simulink library "AC"  (R2020b)
settings: Solver=VariableStepAuto  StartTime=0.0  StopTime=10.0  RelTol=1e-3
undefined symbols (not defined in the file or in its folder): entity, initX, instancedAC, m, n, WP, WPabort, WPspeed
libraries: aerolibactuator x6, $bdroot x1
settings Model: Creator=Rafael.Casado  LastModifiedBy=usuario
settings DataIOCC: ReturnWorkspaceOutputs=off
settings DebuggingCC: ArithmeticOperatorsInVariantConditions=warning
settings SFSimCC: SimUseLocalCustomCode=off  CustomCodeUndefinedFunction=UseInterfaceOnly
settings RTWCC: RTWUseLocalCustomCode=off
settings CodeAppCC: StateflowObjectComments=on

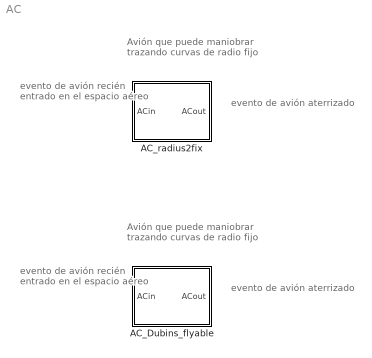
== system AC ==
  note: Avión que puede maniobrar trazando curvas de radio fijo
  note: evento de avión aterrizado
  note: evento de avión recién entrado en el espacio aéreo
  note: Avión que puede maniobrar trazando curvas de radio fijo
  note: evento de avión aterrizado
  note: evento de avión recién entrado en el espacio aéreo
  AC_Dubins_flyable : Subsystem
  AC_radius2fix : Subsystem

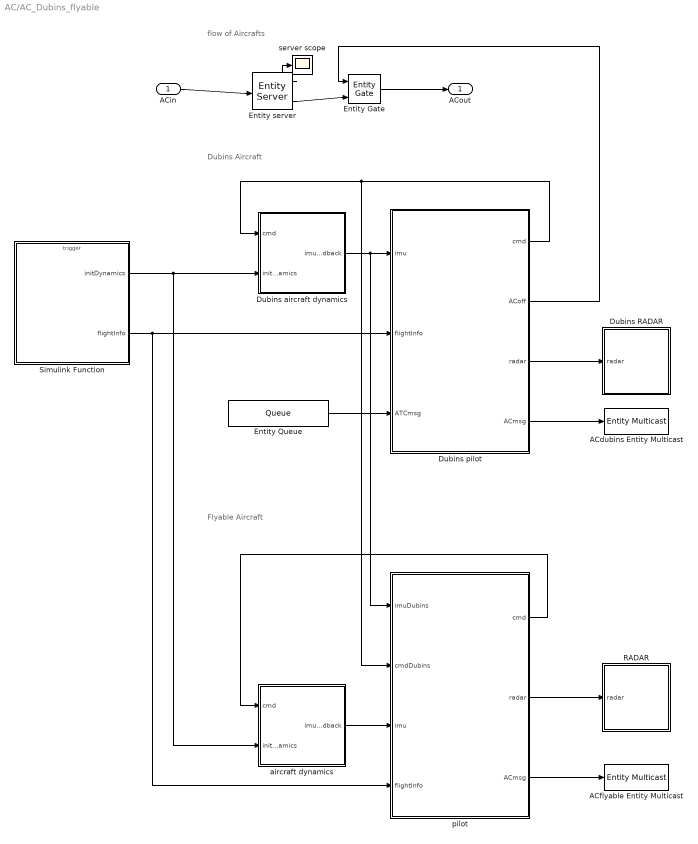
== system AC/AC_Dubins_flyable ==
  note: Dubins Aircraft
  note: flow of Aircrafts
  note: Flyable Aircraft
  ACin : Inport
  ACdubins Entity Multicast : EntityMulticast  InputPortMessageModes=m  MulticastTag=ACcomm
  ACflyable Entity Multicast : EntityMulticast  InputPortMessageModes=m  MulticastTag=ACcomm
  Dubins RADAR : Subsystem
      mask Display:
      | plot([00 10], [05 05])
      | plot([05 05], [00 10])
      | 
      | plot([01 09 09 01 01], [01 01 09 09 01])
      | plot([03 07 07 03 03], [03 03 07 07 03])
  Dubins aircraft dynamics : Subsystem
      mask Display:
      | patch([50 -50 -50 50], [40 40 -60 -60], [1 1 1])
      | 
      | patch([8 -8 -8 8], [6 6 -6 -6], [0.7 0.7 0.7])
      | 
      | patch([ 8  8  28  28], [0 -2 2 4], [0.5 0.5 0.5])
      | patch([-8 -8 -28 -28], [0 -2 2 4], [0.5 0.5 0.5])
      | 
      | patch([1 0 -1], [6 18 6], [0.5 0.5 0.5])
  Dubins pilot : Stateflow chart  TreatAsAtomicUnit=on
  Entity Gate : EntityGate  InputPortMessageModes=m,m  OutputPortMessageModes=m  OperatingMode=Release gate
  Entity Queue : Queue  OutputPortMessageModes=m  Capacity=100  EntityArrivalSource=Multicast  MulticastTag=ATCcomm
  Entity server : EntityServer  InputPortMessageModes=m  OutputPortMessageModes=n,m  Capacity=1  ServiceTimeValue=10  EntryAction=instancedAC(entity.flightId,true);  ServiceCompleteAction=instancedAC(entity.flightId,false);  NumberEntitiesInBlock=on
      settings: OutputPortMap=o1,o9
  RADAR : Subsystem
      mask Display:
      | plot([00 10], [05 05])
      | plot([05 05], [00 10])
      | 
      | plot([01 09 09 01 01], [01 01 09 09 01])
      | plot([03 07 07 03 03], [03 03 07 07 03])
  Simulink Function : Subsystem  TreatAsAtomicUnit=on
  aircraft dynamics : Subsystem
      mask Display:
      | patch([50 -50 -50 50], [40 40 -60 -60], [1 1 1])
      | 
      | patch([8 -8 -8 8], [6 6 -6 -6], [0.7 0.7 0.7])
      | 
      | patch([ 8  8  28  28], [0 -2 2 4], [0.5 0.5 0.5])
      | patch([-8 -8 -28 -28], [0 -2 2 4], [0.5 0.5 0.5])
      | 
      | patch([1 0 -1], [6 18 6], [0.5 0.5 0.5])
  pilot : Stateflow chart  TreatAsAtomicUnit=on
  server scope : Scope
  ACout : Outport  VectorParamsAs1DForOutWhenUnconnected=off
  wires:
  Simulink Function/2(flightInfo) -> pilot/4(flightInfo), Dubins pilot/2(flightInfo)
  ACin/1 -> Entity server/1
  Dubins aircraft dynamics/1(imu_feedback) -> Dubins pilot/1(imu), pilot/1(imuDubins)
  pilot/1(cmd) -> aircraft dynamics/1(cmd)
  Dubins pilot/2(ACoff) -> Entity Gate/1
  pilot/2(radar) -> RADAR/1(radar)
  Simulink Function/1(initDynamics) -> aircraft dynamics/2(initDynamics), Dubins aircraft dynamics/2(initDynamics)
  Dubins pilot/1(cmd) -> pilot/2(cmdDubins), Dubins aircraft dynamics/1(cmd)
  Entity server/1 -> server scope/1
  Dubins pilot/3(radar) -> Dubins RADAR/1(radar)
  aircraft dynamics/1(imu_feedback) -> pilot/3(imu)
  Dubins pilot/4(ACmsg) -> ACdubins Entity Multicast/1
  Entity Gate/1 -> ACout/1
  Entity server/2 -> Entity Gate/2
  Entity Queue/1 -> Dubins pilot/3(ATCmsg)
  pilot/3(ACmsg) -> ACflyable Entity Multicast/1

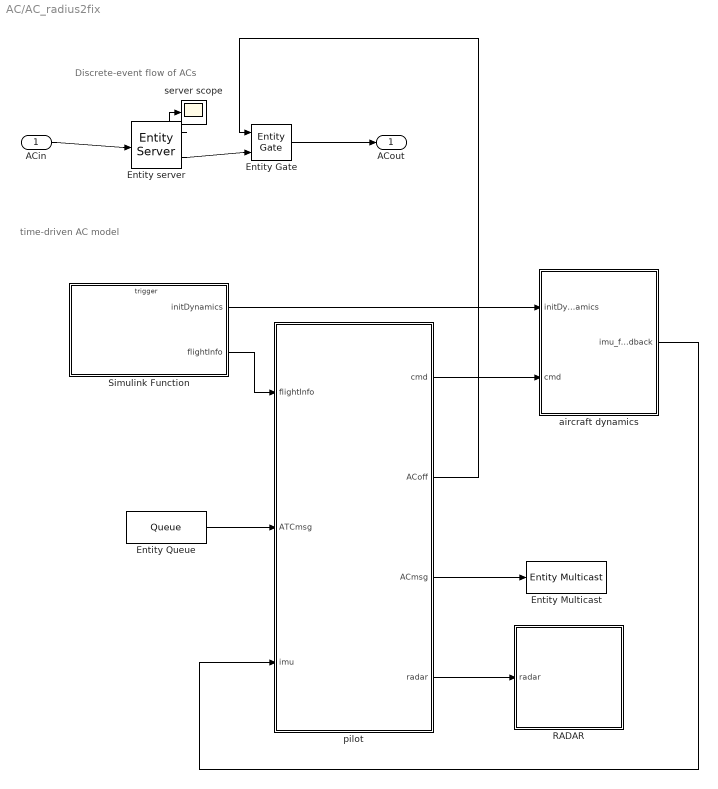
== system AC/AC_radius2fix ==
  note: Discrete-event flow of ACs
  note: time-driven AC model
  ACin : Inport
  Entity Gate : EntityGate  InputPortMessageModes=m,m  OutputPortMessageModes=m  OperatingMode=Release gate
  Entity Multicast : EntityMulticast  InputPortMessageModes=m  MulticastTag=ACcomm
  Entity Queue : Queue  OutputPortMessageModes=m  Capacity=100  EntityArrivalSource=Multicast  MulticastTag=ATCcomm
  Entity server : EntityServer  InputPortMessageModes=m  OutputPortMessageModes=n,m  Capacity=1  ServiceTimeValue=10  EntryAction=instancedAC(entity.flightId,true);  ServiceCompleteAction=instancedAC(entity.flightId,false);  NumberEntitiesInBlock=on
      settings: OutputPortMap=o1,o9
  RADAR : Subsystem
      mask Display:
      | plot([00 10], [05 05])
      | plot([05 05], [00 10])
      | 
      | plot([01 09 09 01 01], [01 01 09 09 01])
      | plot([03 07 07 03 03], [03 03 07 07 03])
  Simulink Function : Subsystem  TreatAsAtomicUnit=on
  aircraft dynamics : Subsystem
      mask Display:
      | patch([50 -50 -50 50], [40 40 -60 -60], [1 1 1])
      | 
      | patch([8 -8 -8 8], [6 6 -6 -6], [0.7 0.7 0.7])
      | 
      | patch([ 8  8  28  28], [0 -2 2 4], [0.5 0.5 0.5])
      | patch([-8 -8 -28 -28], [0 -2 2 4], [0.5 0.5 0.5])
      | 
      | patch([1 0 -1], [6 18 6], [0.5 0.5 0.5])
  pilot : Stateflow chart  TreatAsAtomicUnit=on
  server scope : Scope
  ACout : Outport  VectorParamsAs1DForOutWhenUnconnected=off
  wires:
  aircraft dynamics/1(imu_feedback) -> pilot/3(imu)
  Simulink Function/1(initDynamics) -> aircraft dynamics/1(initDynamics)
  ACin/1 -> Entity server/1
  Simulink Function/2(flightInfo) -> pilot/1(flightInfo)
  Entity Gate/1 -> ACout/1
  Entity server/2 -> Entity Gate/2
  pilot/2(ACoff) -> Entity Gate/1
  pilot/1(cmd) -> aircraft dynamics/2(cmd)
  Entity server/1 -> server scope/1
  pilot/4(radar) -> RADAR/1(radar)
  Entity Queue/1 -> pilot/2(ATCmsg)
  pilot/3(ACmsg) -> Entity Multicast/1

== system AC/AC_Dubins_flyable/Dubins RADAR ==
  radar : Inport
  RADAR figure : MATLABFcn  Commented=on  StartFcn=|  MATLABFcn=PBNsim_RADAR  OutputDimensions=0  Output1D=off
      | clear functions;
      | clc;
      mask Display: patch([50 -50 -50 50], [40 40 -60 -60], [1 1 1])
  virtual bus : Subsystem
  wires:
  radar/1 -> virtual bus/1(nvbus)
  virtual bus/1(vbus) -> RADAR figure/1

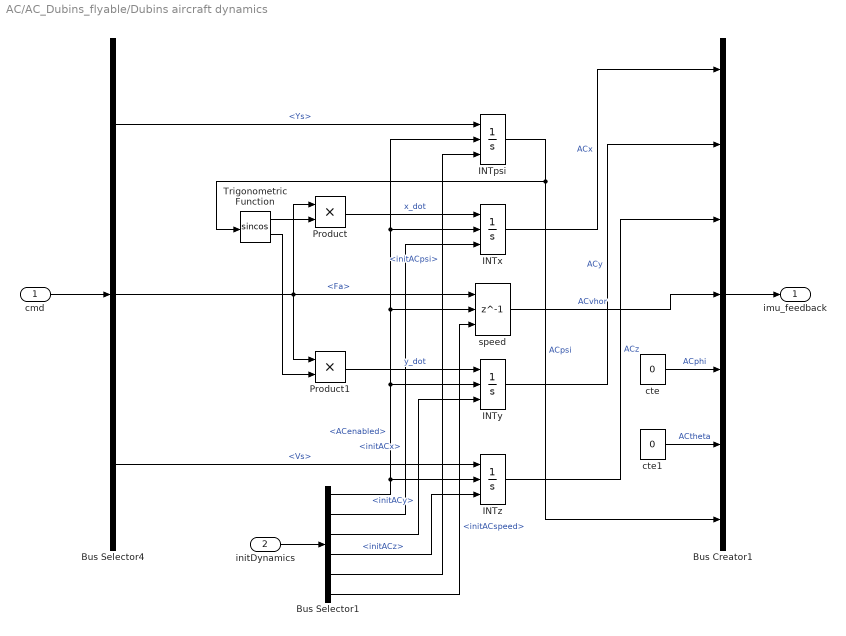
== system AC/AC_Dubins_flyable/Dubins aircraft dynamics ==
  cmd : Inport
  initDynamics : Inport  Port=2
  Bus Creator1 : BusCreator  Inputs=7  OutDataTypeStr=Bus: bus_IMU
      settings: InheritFromInputs=off
  Bus Selector1 : BusSelector  OutputSignals=ACenabled,initACx,initACy,initACz,initACpsi,initACspeed
  Bus Selector4 : BusSelector  OutputSignals=Ys,Fa,Vs
  INTpsi : Integrator  ExternalReset=rising  InitialConditionSource=external  InitialCondition=initX(3)
  INTx : Integrator  ExternalReset=rising  InitialConditionSource=external  InitialCondition=initX(3)
  INTy : Integrator  ExternalReset=rising  InitialConditionSource=external  InitialCondition=initX(3)
  INTz : Integrator  ExternalReset=rising  InitialConditionSource=external  InitialCondition=initX(3)
  Product : Product
  Product1 : Product
  Trigonometric Function : Trigonometry  Operator=sincos
  cte : Constant  Value=0
  cte1 : Constant  Value=0
  speed : Delay  DelayLength=1  InitialConditionSource=Input port  InitialCondition=convvel(240,'kts','m/s');  ExternalReset=Rising
      settings: InputPortMap=u0,r5,p4
  imu_feedback : Outport  SourceOfInitialOutputValue=Input signal  OutputWhenDisabled=reset  VectorParamsAs1DForOutWhenUnconnected=off
  wires:
  Bus Selector4/2 -> Product/1, speed/1, Product1/1  "<Fa>"
  Trigonometric Function/1 -> Product/2
  Product1/1 -> INTy/1  "y_dot"
  Product/1 -> INTx/1  "x_dot"
  Trigonometric Function/2 -> Product1/2
  Bus Selector4/3 -> INTz/1  "<Vs>"
  cmd/1 -> Bus Selector4/1
  Bus Selector4/1 -> INTpsi/1  "<Ys>"
  cte1/1 -> Bus Creator1/6  "ACtheta"
  INTz/1 -> Bus Creator1/3  "ACz"
  INTx/1 -> Bus Creator1/1  "ACx"
  cte/1 -> Bus Creator1/5  "ACphi"
  INTy/1 -> Bus Creator1/2  "ACy"
  Bus Creator1/1 -> imu_feedback/1
  initDynamics/1 -> Bus Selector1/1
  Bus Selector1/2 -> INTx/3  "<initACx>"
  Bus Selector1/3 -> INTy/3  "<initACy>"
  Bus Selector1/4 -> INTz/3  "<initACz>"
  Bus Selector1/5 -> INTpsi/3  "<initACpsi>"
  Bus Selector1/1 -> INTz/2, speed/2, INTpsi/2, INTx/2, INTy/2  "<ACenabled>"
  INTpsi/1 -> Bus Creator1/7, Trigonometric Function/1  "ACpsi"
  speed/1 -> Bus Creator1/4  "ACvhor"
  Bus Selector1/6 -> speed/3  "<initACspeed>"

== system AC/AC_Dubins_flyable/RADAR ==
  radar : Inport
  RADAR figure : MATLABFcn  StartFcn=|  MATLABFcn=PBNsim_RADAR  OutputDimensions=0  Output1D=off
      | clear functions;
      | clc;
      mask Display: patch([50 -50 -50 50], [40 40 -60 -60], [1 1 1])
  virtual bus : $bdroot/AC_Dubins_flyable/Dubins RADAR/virtual bus  SystemSampleTime=-1  VariantActivationTime=update diagram  Latency=0  AutoFrameSizeCalculation=off
  wires:
  radar/1 -> virtual bus/1
  virtual bus/1 -> RADAR figure/1

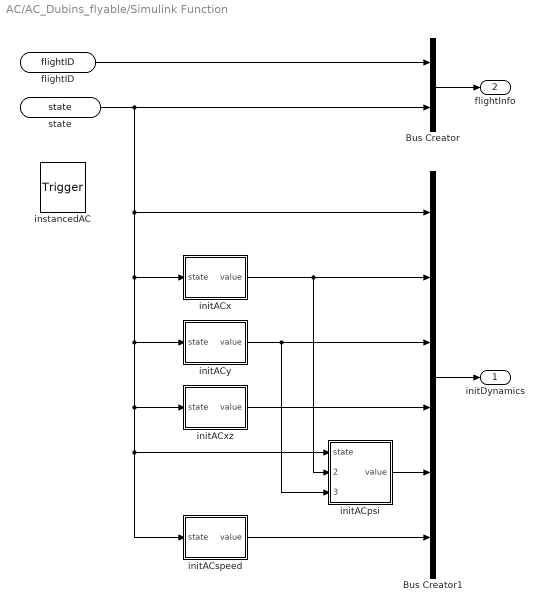
== system AC/AC_Dubins_flyable/Simulink Function ==
  instancedAC : TriggerPort  TriggerType=function-call  IsSimulinkFunction=on  FunctionName=instancedAC  FunctionVisibility=scoped  VariantControl=Variant
  Bus Creator : BusCreator  Inputs=2  OutDataTypeStr=Bus: bus_ADSB
      settings: InheritFromInputs=off
  Bus Creator1 : BusCreator  Inputs=6  OutDataTypeStr=Bus: bus_initDynamics
      settings: InheritFromInputs=off
  initACpsi : Subsystem
  initACspeed : Subsystem
  initACx : Subsystem
  initACxz : Subsystem
  initACy : Subsystem
  flightID : ArgIn  ArgumentName=flightID
  state : ArgIn  Port=2  OutDataTypeStr=boolean  ArgumentName=state
  initDynamics : Outport  VectorParamsAs1DForOutWhenUnconnected=off
  flightInfo : Outport  Port=2  VectorParamsAs1DForOutWhenUnconnected=off
  wires:
  state/1 -> initACy/1(state), initACxz/1(state), initACpsi/1(state), initACspeed/1(state), initACx/1(state), Bus Creator1/1, Bus Creator/2
  Bus Creator/1 -> flightInfo/1
  flightID/1 -> Bus Creator/1
  Bus Creator1/1 -> initDynamics/1
  initACx/1(value) -> initACpsi/2(initACx), Bus Creator1/2
  initACy/1(value) -> initACpsi/3(initACy), Bus Creator1/3
  initACxz/1(value) -> Bus Creator1/4
  initACpsi/1(value) -> Bus Creator1/5
  initACspeed/1(value) -> Bus Creator1/6

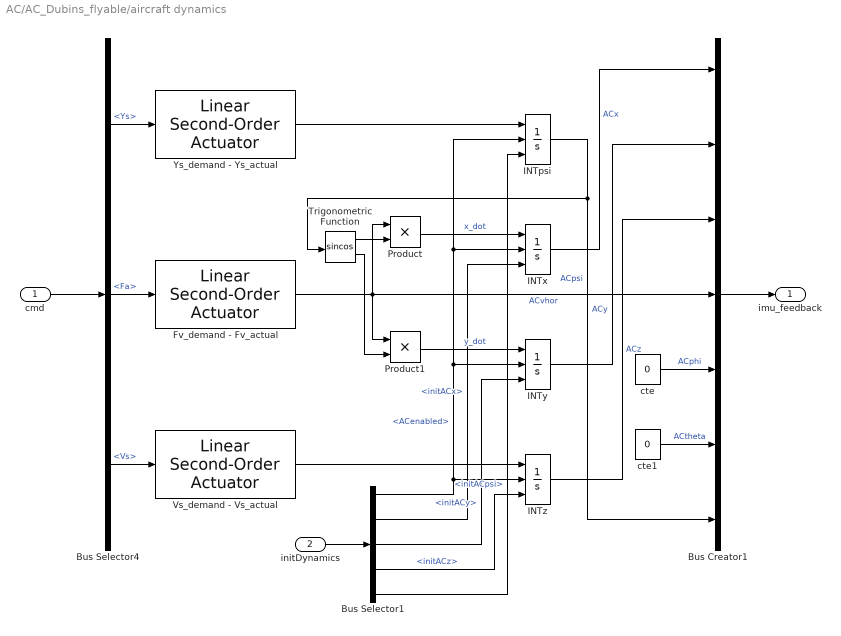
== system AC/AC_Dubins_flyable/aircraft dynamics ==
  cmd : Inport
  initDynamics : Inport  Port=2
  Bus Creator1 : BusCreator  Inputs=7  OutDataTypeStr=Bus: bus_IMU
      settings: InheritFromInputs=off
  Bus Selector1 : BusSelector  OutputSignals=ACenabled,initACx,initACy,initACz,initACpsi
  Bus Selector4 : BusSelector  OutputSignals=Ys,Fa,Vs
  Fv_demand - Fv_actual : aerolibactuator/Linear Second-Order Actuator  wn_fin=0.6  z_fin=1  fin_act_0=convvel(240,'kts','m/s');  fin_act_vel=0
      settings: SourceProductBaseCode=AE
  INTpsi : Integrator  ExternalReset=rising  InitialConditionSource=external  InitialCondition=initX(3)
  INTx : Integrator  ExternalReset=rising  InitialConditionSource=external  InitialCondition=initX(3)
  INTy : Integrator  ExternalReset=rising  InitialConditionSource=external  InitialCondition=initX(3)
  INTz : Integrator  ExternalReset=rising  InitialConditionSource=external  InitialCondition=initX(3)
  Product : Product
  Product1 : Product
  Trigonometric Function : Trigonometry  Operator=sincos
  Vs_demand - Vs_actual : aerolibactuator/Linear Second-Order Actuator  wn_fin=0.6  z_fin=1  fin_act_0=0  fin_act_vel=0
      settings: SourceProductBaseCode=AE
  Ys_demand - Ys_actual : aerolibactuator/Linear Second-Order Actuator  wn_fin=0.8  z_fin=1  fin_act_0=0  fin_act_vel=0
      settings: SourceProductBaseCode=AE
  cte : Constant  Value=0
  cte1 : Constant  Value=0
  imu_feedback : Outport  SourceOfInitialOutputValue=Input signal  OutputWhenDisabled=reset  VectorParamsAs1DForOutWhenUnconnected=off
  wires:
  Bus Selector4/2 -> Fv_demand - Fv_actual/1  "<Fa>"
  Fv_demand - Fv_actual/1 -> Product/1, Product1/1, Bus Creator1/4  "ACvhor"
  Trigonometric Function/1 -> Product/2
  Product1/1 -> INTy/1  "y_dot"
  Product/1 -> INTx/1  "x_dot"
  Trigonometric Function/2 -> Product1/2
  Bus Selector4/3 -> Vs_demand - Vs_actual/1  "<Vs>"
  cmd/1 -> Bus Selector4/1
  Bus Selector4/1 -> Ys_demand - Ys_actual/1  "<Ys>"
  cte1/1 -> Bus Creator1/6  "ACtheta"
  INTz/1 -> Bus Creator1/3  "ACz"
  INTx/1 -> Bus Creator1/1  "ACx"
  cte/1 -> Bus Creator1/5  "ACphi"
  INTy/1 -> Bus Creator1/2  "ACy"
  Bus Creator1/1 -> imu_feedback/1
  initDynamics/1 -> Bus Selector1/1
  Bus Selector1/2 -> INTx/3  "<initACx>"
  Bus Selector1/3 -> INTy/3  "<initACy>"
  Bus Selector1/4 -> INTz/3  "<initACz>"
  Bus Selector1/5 -> INTpsi/3  "<initACpsi>"
  Bus Selector1/1 -> INTz/2, INTpsi/2, INTx/2, INTy/2  "<ACenabled>"
  INTpsi/1 -> Trigonometric Function/1, Bus Creator1/7  "ACpsi"
  Vs_demand - Vs_actual/1 -> INTz/1
  Ys_demand - Ys_actual/1 -> INTpsi/1

== system AC/AC_radius2fix/RADAR ==
  radar : Inport
  RADAR figure : MATLABFcn  StartFcn=|  MATLABFcn=PBNsim_RADAR  OutputDimensions=0  Output1D=off
      | clear functions;
      | clc;
      mask Display: patch([50 -50 -50 50], [40 40 -60 -60], [1 1 1])
  virtual bus : Subsystem
  wires:
  radar/1 -> virtual bus/1(nvbus)
  virtual bus/1(vbus) -> RADAR figure/1

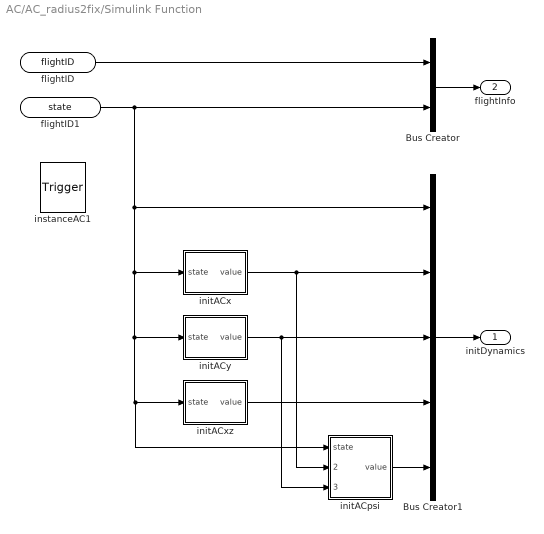
== system AC/AC_radius2fix/Simulink Function ==
  instanceAC1 : TriggerPort  TriggerType=function-call  IsSimulinkFunction=on  FunctionName=instancedAC  FunctionVisibility=scoped  VariantControl=Variant
  Bus Creator : BusCreator  Inputs=2  OutDataTypeStr=Bus: bus_ADSB
      settings: InheritFromInputs=off
  Bus Creator1 : BusCreator  Inputs=5  OutDataTypeStr=Bus: bus_initDynamics
      settings: InheritFromInputs=off
  initACpsi : Subsystem
  initACx : Subsystem
  initACxz : Subsystem
  initACy : Subsystem
  flightID : ArgIn  ArgumentName=flightID
  flightID1 : ArgIn  Port=2  OutDataTypeStr=boolean  ArgumentName=state
  initDynamics : Outport  VectorParamsAs1DForOutWhenUnconnected=off
  flightInfo : Outport  Port=2  VectorParamsAs1DForOutWhenUnconnected=off
  wires:
  initACpsi/1(value) -> Bus Creator1/5
  initACxz/1(value) -> Bus Creator1/4
  initACy/1(value) -> initACpsi/3(initACy), Bus Creator1/3
  initACx/1(value) -> Bus Creator1/2, initACpsi/2(initACx)
  Bus Creator1/1 -> initDynamics/1
  flightID/1 -> Bus Creator/1
  Bus Creator/1 -> flightInfo/1
  flightID1/1 -> Bus Creator/2, initACx/1(state), initACxz/1(state), initACpsi/1(state), initACy/1(state), Bus Creator1/1

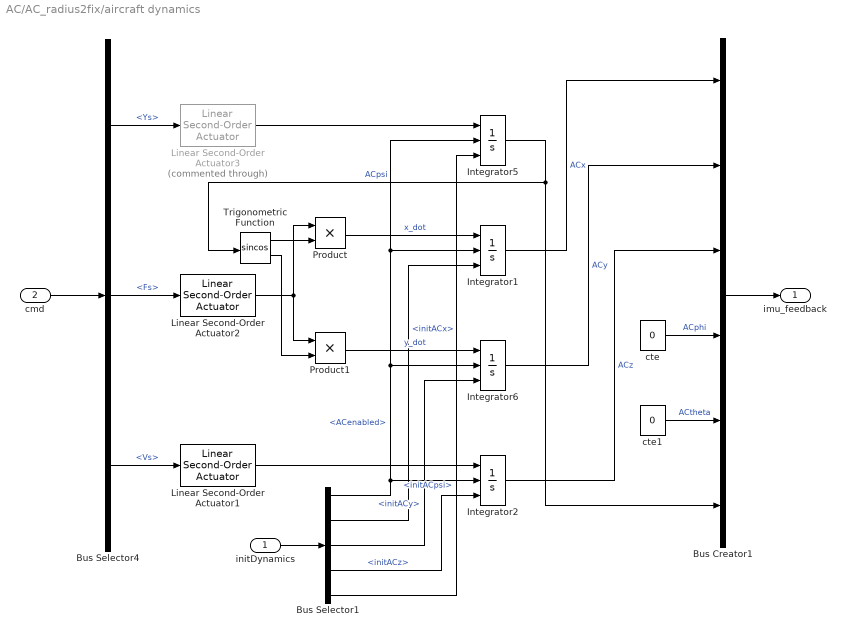
== system AC/AC_radius2fix/aircraft dynamics ==
  initDynamics : Inport
  cmd : Inport  Port=2
  Bus Creator1 : BusCreator  Inputs=6  OutDataTypeStr=Bus: bus_IMU
      settings: InheritFromInputs=off
  Bus Selector1 : BusSelector  OutputSignals=ACenabled,initACx,initACy,initACz,initACpsi
  Bus Selector4 : BusSelector  OutputSignals=Ys,Fs,Vs
  Integrator{1..2,5..6} (4 alike) : Integrator  ExternalReset=rising  InitialConditionSource=external  InitialCondition=initX(3)
  Linear Second-Order Actuator1 : aerolibactuator/Linear Second-Order Actuator  wn_fin=1  z_fin=1  fin_act_0=0  fin_act_vel=0
      settings: SourceProductBaseCode=AE
  Linear Second-Order Actuator2 : aerolibactuator/Linear Second-Order Actuator  wn_fin=1  z_fin=1  fin_act_0=convvel(240,'kts','m/s');  fin_act_vel=0
      settings: SourceProductBaseCode=AE
  Linear Second-Order Actuator3 : aerolibactuator/Linear Second-Order Actuator  Commented=through  wn_fin=1  z_fin=1  fin_act_0=0  fin_act_vel=0
      settings: SourceProductBaseCode=AE
  Product : Product
  Product1 : Product
  Trigonometric Function : Trigonometry  Operator=sincos
  cte : Constant  Value=0
  cte1 : Constant  Value=0
  imu_feedback : Outport  SourceOfInitialOutputValue=Input signal  OutputWhenDisabled=reset  VectorParamsAs1DForOutWhenUnconnected=off
  wires:
  Integrator5/1 -> Bus Creator1/6, Trigonometric Function/1  "ACpsi"
  Bus Selector1/1 -> Integrator2/2, Integrator6/2, Integrator1/2, Integrator5/2  "<ACenabled>"
  Bus Selector1/5 -> Integrator5/3  "<initACpsi>"
  Bus Selector1/4 -> Integrator2/3  "<initACz>"
  Bus Selector1/3 -> Integrator6/3  "<initACy>"
  Bus Selector1/2 -> Integrator1/3  "<initACx>"
  initDynamics/1 -> Bus Selector1/1
  Bus Creator1/1 -> imu_feedback/1
  Integrator6/1 -> Bus Creator1/2  "ACy"
  cte/1 -> Bus Creator1/4  "ACphi"
  Integrator1/1 -> Bus Creator1/1  "ACx"
  Integrator2/1 -> Bus Creator1/3  "ACz"
  cte1/1 -> Bus Creator1/5  "ACtheta"
  Bus Selector4/1 -> Linear Second-Order Actuator3/1  "<Ys>"
  cmd/1 -> Bus Selector4/1
  Bus Selector4/3 -> Linear Second-Order Actuator1/1  "<Vs>"
  Trigonometric Function/2 -> Product1/2
  Product/1 -> Integrator1/1  "x_dot"
  Bus Selector4/2 -> Linear Second-Order Actuator2/1  "<Fs>"
  Product1/1 -> Integrator6/1  "y_dot"
  Trigonometric Function/1 -> Product/2
  Linear Second-Order Actuator2/1 -> Product/1, Product1/1
  Linear Second-Order Actuator1/1 -> Integrator2/1
  Linear Second-Order Actuator3/1 -> Integrator5/1

== system AC/AC_Dubins_flyable/Dubins RADAR/virtual bus ==
  nvbus : Inport
  Bus Creator : BusCreator  Inputs=7  OutDataTypeStr=Bus: bus_radar
      settings: InheritFromInputs=off
  Bus Selector4 : BusSelector  OutputSignals=ACid,ACenabled,ACdubins,ACx,ACy,ACz,ACpsi
  vbus : Outport  VectorParamsAs1DForOutWhenUnconnected=off
  wires:
  Bus Selector4/1 -> Bus Creator/1  "<ACid>"
  Bus Selector4/4 -> Bus Creator/4  "<ACx>"
  Bus Selector4/6 -> Bus Creator/6  "<ACz>"
  Bus Selector4/5 -> Bus Creator/5  "<ACy>"
  Bus Selector4/2 -> Bus Creator/2  "<ACenabled>"
  nvbus/1 -> Bus Selector4/1
  Bus Creator/1 -> vbus/1
  Bus Selector4/3 -> Bus Creator/3  "<ACdubins>"
  Bus Selector4/7 -> Bus Creator/7  "<ACpsi>"

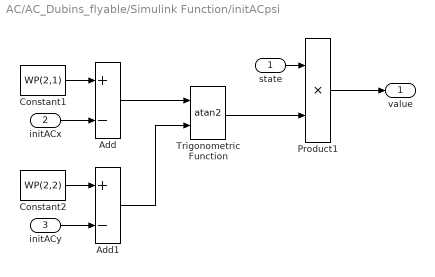
== system AC/AC_Dubins_flyable/Simulink Function/initACpsi ==
  state : Inport
  initACx : Inport  Port=2
  initACy : Inport  Port=3
  Add : Sum  Inputs=+-
  Add1 : Sum  Inputs=+-
  Constant1 : Constant  Value=WP(2,1)
  Constant2 : Constant  Value=WP(2,2)
  Product1 : Product
  Trigonometric Function : Trigonometry  Operator=atan2
  value : Outport  VectorParamsAs1DForOutWhenUnconnected=off
  wires:
  Add1/1 -> Trigonometric Function/2
  Add/1 -> Trigonometric Function/1
  Constant2/1 -> Add1/1
  initACy/1 -> Add1/2
  initACx/1 -> Add/2
  Constant1/1 -> Add/1
  state/1 -> Product1/1
  Trigonometric Function/1 -> Product1/2
  Product1/1 -> value/1

== system AC/AC_Dubins_flyable/Simulink Function/initACspeed ==
  state : Inport
  Add : Sum
  Constant1 : Constant  Value=convvel(WPspeed(2),'kts','m/s');
  Product1 : Product
  Uniform Random Number : UniformRandomNumber  Commented=on  Minimum=0  Maximum=100  Seed=randi(10000)
  value : Outport  VectorParamsAs1DForOutWhenUnconnected=off
  wires:
  Add/1 -> Product1/2
  Constant1/1 -> Add/1
  state/1 -> Product1/1
  Product1/1 -> value/1
  Uniform Random Number/1 -> Add/2

== system AC/AC_Dubins_flyable/Simulink Function/initACx ==
  state : Inport
  Add : Sum
  Constant1 : Constant  Value=WP(1,1)
  Product1 : Product
  Uniform Random Number : UniformRandomNumber  Commented=on  Minimum=0  Maximum=100  Seed=randi(10000)
  value : Outport  VectorParamsAs1DForOutWhenUnconnected=off
  wires:
  Add/1 -> Product1/2
  Constant1/1 -> Add/1
  state/1 -> Product1/1
  Product1/1 -> value/1
  Uniform Random Number/1 -> Add/2

== system AC/AC_Dubins_flyable/Simulink Function/initACxz ==
  state : Inport
  Add1 : Sum
  Constant2 : Constant  Value=WP(1,3)
  Product1 : Product
  Uniform Random Number1 : UniformRandomNumber  Commented=on  Minimum=0  Maximum=20  Seed=randi(10000)
  value : Outport  VectorParamsAs1DForOutWhenUnconnected=off
  wires:
  Uniform Random Number1/1 -> Add1/2
  Add1/1 -> Product1/2
  Constant2/1 -> Add1/1
  state/1 -> Product1/1
  Product1/1 -> value/1

== system AC/AC_Dubins_flyable/Simulink Function/initACy ==
  state : Inport
  Add2 : Sum
  Constant1 : Constant  Value=WP(1,2)
  Product1 : Product
  Uniform Random Number2 : UniformRandomNumber  Commented=on  Minimum=0  Maximum=100  Seed=randi(10000)
  value : Outport  VectorParamsAs1DForOutWhenUnconnected=off
  wires:
  Constant1/1 -> Add2/1
  Add2/1 -> Product1/2
  Uniform Random Number2/1 -> Add2/2
  state/1 -> Product1/1
  Product1/1 -> value/1

== system AC/AC_radius2fix/RADAR/virtual bus ==
  nvbus : Inport
  Bus Creator : BusCreator  Inputs=6  OutDataTypeStr=Bus: bus_radar
      settings: InheritFromInputs=off
  Bus Selector4 : BusSelector  OutputSignals=ACid,ACenabled,ACx,ACy,ACz,ACpsi
  vbus : Outport  VectorParamsAs1DForOutWhenUnconnected=off
  wires:
  Bus Creator/1 -> vbus/1
  nvbus/1 -> Bus Selector4/1
  Bus Selector4/2 -> Bus Creator/2  "<ACenabled>"
  Bus Selector4/4 -> Bus Creator/4  "<ACy>"
  Bus Selector4/6 -> Bus Creator/6  "<ACpsi>"
  Bus Selector4/5 -> Bus Creator/5  "<ACz>"
  Bus Selector4/3 -> Bus Creator/3  "<ACx>"
  Bus Selector4/1 -> Bus Creator/1  "<ACid>"

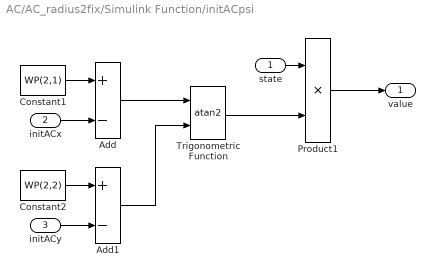
== system AC/AC_radius2fix/Simulink Function/initACpsi ==
  state : Inport
  initACx : Inport  Port=2
  initACy : Inport  Port=3
  Add : Sum  Inputs=+-
  Add1 : Sum  Inputs=+-
  Constant1 : Constant  Value=WP(2,1)
  Constant2 : Constant  Value=WP(2,2)
  Product1 : Product
  Trigonometric Function : Trigonometry  Operator=atan2
  value : Outport  VectorParamsAs1DForOutWhenUnconnected=off
  wires:
  Product1/1 -> value/1
  Trigonometric Function/1 -> Product1/2
  state/1 -> Product1/1
  Constant1/1 -> Add/1
  initACx/1 -> Add/2
  initACy/1 -> Add1/2
  Constant2/1 -> Add1/1
  Add/1 -> Trigonometric Function/1
  Add1/1 -> Trigonometric Function/2

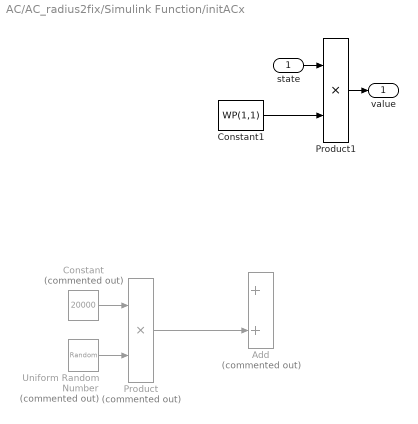
== system AC/AC_radius2fix/Simulink Function/initACx ==
  state : Inport
  Add : Sum  Commented=on
  Constant : Constant  Commented=on  Value=20000
  Constant1 : Constant  Value=WP(1,1)
  Product : Product  Commented=on
  Product1 : Product
  Uniform Random Number : UniformRandomNumber  Commented=on  Minimum=0  Seed=randi(10000)
  value : Outport  VectorParamsAs1DForOutWhenUnconnected=off
  wires:
  Constant/1 -> Product/1
  Uniform Random Number/1 -> Product/2
  Product/1 -> Add/2
  Product1/1 -> value/1
  state/1 -> Product1/1
  Constant1/1 -> Product1/2

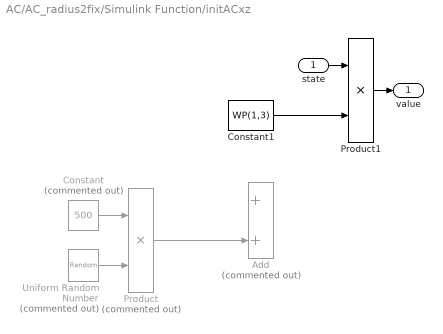
== system AC/AC_radius2fix/Simulink Function/initACxz ==
  state : Inport
  Add : Sum  Commented=on
  Constant : Constant  Commented=on  Value=500
  Constant1 : Constant  Value=WP(1,3)
  Product : Product  Commented=on
  Product1 : Product
  Uniform Random Number : UniformRandomNumber  Commented=on  Minimum=0  Seed=randi(10000)
  value : Outport  VectorParamsAs1DForOutWhenUnconnected=off
  wires:
  Constant/1 -> Product/1
  Uniform Random Number/1 -> Product/2
  Product/1 -> Add/2
  Product1/1 -> value/1
  Constant1/1 -> Product1/2
  state/1 -> Product1/1

== system AC/AC_radius2fix/Simulink Function/initACy ==
  state : Inport
  Add : Sum  Commented=on
  Constant : Constant  Commented=on  Value=20000
  Constant1 : Constant  Value=WP(1,2)
  Product : Product  Commented=on
  Product1 : Product
  Uniform Random Number : UniformRandomNumber  Commented=on  Minimum=0  Seed=randi(10000)
  value : Outport  VectorParamsAs1DForOutWhenUnconnected=off
  wires:
  Constant/1 -> Product/1
  Uniform Random Number/1 -> Product/2
  Product/1 -> Add/2
  Product1/1 -> value/1
  Constant1/1 -> Product1/2
  state/1 -> Product1/1

== stateflow chart AC/AC_radius2fix/pilot ==
  state NAVIGATOR [parallel]
    settings: executionOrder=1
    state OFF
      entry:
      ACid = 0;
      ACenabled = 0;
      cmd.Fs = 123; %m/s
    state ON
      entry:
      initAC;
      ACmsgSend;
    state FLYING
      entry, during:
      fly;
      ACmsgSend;
    state LANDED
      entry:
      landed;
      ACoff.data = true;
      send(ACoff);
      ACmsgSend;
    (default) -> OFF
    OFF -> ON : [flightInfo.ACenabled]
    LANDED -> OFF
    ON -> FLYING
    FLYING -> LANDED [order 1] : [landedAC]
    FLYING -> FLYING [order 2] : [abortLanding]
  state COMUNICATIONS [parallel]
    updateRadar
    msgProcess
    settings: executionOrder=2
    state msgProcess [function]
      (default) -> (junction 143)
      (junction 143) -> (junction 138) [order 1] : ATCmsg
      (junction 145) -> (junction 143)
      (junction 143) -> (junction 139) [order 2]
      (junction 138) -> (junction 145) : {ATCmsgProcess}
  data: landed function_output; abort function_output; cmd output Bus: bus_command; flightInfo input Bus: bus_ADSB; ATCmsg input; ACoff output; ACmsg output Bus: bus_ACmsg; radar output Bus: bus_radar; ACid local double; imu input; cWP local; dist local; WP parameter; WPabort parameter; WPspeed parameter; ACenabled local; ACaborted local
  function initAC:
    | function initAC
    | 
    | % Inicializo identificador del avion
    | ACid = flightInfo.ACid;
    | ACenabled = 1;
    | ACaborted = 0;
    | 
    | % Inicializo bus de comandos
    | coder.extrinsic('convvel');
    | cmd.Fs = convvel(240,'kts','m/s'); %123 m/s
    | cmd.Vs = 0;
    | cmd.Ys = 0;
    | 
    | % inicializo navegación
    | cWP = [WP(2,:) WPspeed(2)];
  function landed = landedAC:
    | function landed = landedAC
    | % Concluye si el avion ha terminado de recorrer la pista
    | 
    | landed = false;
    | threshold = 5;
    | if abs(cWP(4) - 50) < threshold % la velocidad a 50 solo la tiene el último waypoint
    | % if cWP(4) == 50 % la velocidad a 50 solo la tiene el último waypoint
    |     %calculo segmento desde el AC a este WP
    |     s = cWP(1:2)-[imu.ACx imu.ACy];
    |     dist = norm(s);
    |     if dist < 50
    |         landed = true;
    |     end
    | end
  function fly:
    | function fly
    | 
    | % radio de giro
    | r = 2815; % convlength(1.52,'naut mi','m')
    | 
    | 
    | %calculo vector AC -> WP actual
    | vec_AC_cWP = cWP(1:2)-[imu.ACx imu.ACy];
    | dist = norm(vec_AC_cWP);
    | 
    | 
    | 
    | %calculo vector AC->dirAC
    | vec_AC_dir = [sin(imu.ACpsi) cos(imu.ACpsi)];
    | 
    | 
    | %determino si el giro es a izquierda o derecha
    | izqder = vec_AC_dir(1)*vec_AC_cWP(2) - vec_AC_dir(2)*vec_AC_cWP(1);
    | 
    | if izqder > 0
    |     cmd.Ys = -cmd.Fs/r;
    | elseif izqder < 0
    |     cmd.Ys = +cmd.Fs/r;
    | else
    |     cmd.Ys = 0;
    | end
    | 
    | 
    | %calculo velocidad vertical
    | dist_vertical = cWP(3) - imu.ACz;
    | tiempo = dist / cmd.Fs;
    | cmd.Vs = dist_vertical / tiempo;
    | 
    | %establezco velocidad horizontal
    | coder.extrinsic('convvel');
    | cmd.Fs = convvel(cWP(4),'kts','m/s'); %123 m/s
  function landed:
    | function landed
    | cmd.Fs = 0;
    | cmd.Vs = 0;
    | cmd.Ys = 0;
    | ACenabled = 0;
  function abort = abortLanding:
    | function abort = abortLanding
    | % Decido si abortar el aterrizaje
    | % 
    | % persistent previously_aborted 
    | % if isempty(previously_aborted)
    | %     previously_aborted = false;
    | % end
    | 
    | abort = false;
    | 
    | if ACaborted
    |     return
    | end
    | 
    | if (ACid == 5) && (imu.ACz < 90) % DA/H: 295 ft (89.9 m)
    |     abort = true;
    |     ACaborted = 1;
    | %    cWP = [WP(WPabort,:) WPspeed(WPabort)];
    | end
  function ACmsgSend:
    | function ACmsgSend
    | ACmsg.ACid      = ACid;
    | ACmsg.ACenabled = ACenabled;
    | ACmsg.ACx       = imu.ACx;
    | ACmsg.ACy       = imu.ACy;
    | ACmsg.ACz       = imu.ACz;
    | ACmsg.ACpsi     = imu.ACpsi;
    | ACmsg.ACaborted = ACaborted;
    | send(ACmsg)
  function updateRadar:
    | function updateRadar
    | 
    | radar.ACid      = ACid;
    | radar.ACenabled = ACenabled;
    | radar.ACx       = imu.ACx;
    | radar.ACy       = imu.ACy;
    | radar.ACz       = imu.ACz;
    | radar.ACpsi     = imu.ACpsi;
  function ATCmsgProcess:
    | function ATCmsgProcess
    | 
    | % extraigo informacion del mensaje
    | if ACenabled && ACid == ATCmsg.ACid
    |         cWP = [ATCmsg.WPx ATCmsg.WPy ATCmsg.WPz ATCmsg.WPspeed];
    | end
    | discard(ATCmsg)
    | 
    | %% Procesamiento del ATC

== stateflow chart AC/AC_Dubins_flyable/Dubins pilot ==
  state NAVIGATOR [parallel]
    settings: executionOrder=1
    state OFF
      entry:
      reset
    state ON
      entry:
      wakeUp
      ACmsgSend
    state FLYING
      entry, during:
      fly
      ACmsgSend
    state SLEEP
      entry:
      sleep
      ACmsgSend
    (default) -> OFF
    OFF -> ON : [flightInfo.ACenabled]
    ON -> FLYING
    SLEEP -> OFF
    FLYING -> SLEEP [order 1] : [landedAC]
    FLYING -> FLYING [order 2] : [abortLanding]
  state COMUNICATIONS [parallel]
    updateRadar
    msgProcess
    settings: executionOrder=2
    state msgProcess [function]
      (default) -> (junction 143)
      (junction 143) -> (junction 138) [order 1] : ATCmsg
      (junction 145) -> (junction 143)
      (junction 143) -> (junction 139) [order 2]
      (junction 138) -> (junction 145) : {ATCmsgProcess}
  data: landed function_output; abort function_output; imu input; cmd output Bus: bus_command; flightInfo input Bus: bus_ADSB; ATCmsg input; ACoff output; radar output Bus: bus_radar; ACmsg output Bus: bus_ACmsg; ACid local double; cWP local; dist local; WP parameter; WPspeed parameter; ACenabled local; ACaborted local
  function reset:
    | function reset
    | 
    | % reseteo estado de la aeronave
    | ACid = 0;
    | ACenabled = 0;
    | ACaborted = 0;
    | 
    | % reseteo movimiento
    | coder.extrinsic('convvel');
    | cmd.Fa = 123.4667; %convvel(cWP(4),'kts','m/s'); %123 m/s
    | cmd.Vs = 0;
    | cmd.Ys = 0;
  function wakeUp:
    | function wakeUp
    | 
    | % inicializo navegación
    | ACid = flightInfo.ACid;
    | ACenabled = 1;
    | cWP = [WP(2,:) WPspeed(2)];
  function landed = landedAC:
    | function landed = landedAC
    | % Concluye si el avion ha terminado de recorrer la pista
    | 
    | landed = false;
    | 
    | if cWP(4) == 50 % la velocidad a 50 solo la tiene el último waypoint
    |     %calculo segmento desde el AC a este WP
    |     s = cWP(1:2)-[imu.ACx imu.ACy];
    |     dist = norm(s);
    |     if dist < 50
    |         landed = true;
    |     end
    | end
  function fly:
    | function fly
    | 
    | % radio de giro
    | r = 2815; % convlength(1.52,'naut mi','m')
    | 
    | %calculo vector AC -> WP actual
    | vec_ac_wp = cWP(1:2) - [imu.ACx imu.ACy];
    | dis_ac_wp = norm(vec_ac_wp);
    | 
    | 
    | %calculo vector AC->dirAC
    | vec_ac_dir = [sin(imu.ACpsi) cos(imu.ACpsi)];
    | 
    | 
    | %determino si el giro es a izquierda o derecha, y el angulo
    | ang_dir_wp = angulo(vec_ac_dir,vec_ac_wp);
    | 
    | 
    | %giramos hacia el lado correcto
    | if ang_dir_wp > 0
    |     % giramos a babor (izquierda)
    |     cmd.Ys = -imu.ACvhor/r;
    |     vec_cc_ac = [sin(imu.ACpsi+pi/2) cos(imu.ACpsi+pi/2)];
    | elseif ang_dir_wp < 0
    |     % giramos a estribor (derecha)
    |     cmd.Ys = +imu.ACvhor/r;
    |     vec_cc_ac = [sin(imu.ACpsi-pi/2) cos(imu.ACpsi-pi/2)];
    | else
    |     % seguimos recto
    |     cmd.Ys = 0;
    |     vec_cc_ac = vec_ac_dir;
    | end
    | 
    | 
    | if ang_dir_wp == 0
    |     dis_hor = dis_ac_wp;
    | else
    | 
    |     %calculo centro de circunferencia de giro
    |     cc = [imu.ACx imu.ACy] - vec_cc_ac * r;
    | 
    |     %compruebo si hay espacio para hacer la curva
    |     vec_cc_wp = cWP(1:2) - cc;
    |     dis_cc_wp = norm(vec_cc_wp);
    |     
    |     if dis_cc_wp < r
    |         % no hay espacio: asumimos recta
    |         dis_hor = dis_ac_wp;
    |     else
    |         %calculo distancia recorrida en linea recta
    |         dis_tc_wp = sqrt(dis_cc_wp^2 - r^2);
    | 
    |         %calculo distancia recorrida en linea curva
    |         ang_cc_tc = atand(r/dis_tc_wp);
    |         ang_tc_wp = 90 - ang_cc_tc;
    |         ang_ac_wp = angulo(vec_cc_ac,vec_cc_wp);
    | 
    |         ang_ac_tc = ang_ac_wp - ang_tc_wp;    
    | 
    |         if sign(ang_dir_wp) == sign(ang_ac_wp)
    |             % tienen el mismo signo: por lo que se gira menos de 1/4 de vuelta
    |             ang_ac_tc = abs(ang_ac_wp) - ang_tc_wp;
    |         else
    |             % tienen signo contrario: por lo que se gira mas de 1/4 de vuelta
    |             ang_ac_tc = 360 - abs(ang_ac_wp) - ang_tc_wp;    
    |         end
    | 
    |         dis_ac_tc = deg2rad(ang_ac_tc) * r;
    | 
    |         %calculo distancia horizontal total a recorrer
    |         dis_hor = dis_ac_tc + dis_tc_wp;         
    |         
    |     end
    |     
    | end
    | 
    | 
    | 
    | vwp    = 0;
    | coder.extrinsic('convvel');
    | vwp    = convvel(cWP(4),'kts','m/s'); %123 m/s
    | 
    | %%
    | % modelo de avion que se adapta a la velocidad del nuevo waypoint 
    | % lo mas rapido posible 
    | cmd.Fa = vwp; %usamos el bus de aceleracion para poner la velocidad deseada
    | 
    | %calculo velocidad vertical
    | dis_vertical = cWP(3) - imu.ACz;
    | tiempo = dis_hor / vwp;
    | cmd.Vs = dis_vertical / tiempo;
    | 
    | 
    | 
    | 
    | 
    | 
    | %%
    | % % modelo de avion que se adapta a la velocidad del nuevo waypoint 
    | % % de manera progresiva en el espacio disponible.
    | % % establece aceleración horizontal al despejar el sistema de ecuaciones:
    | % %    v =  v0 + a * t
    | % %    s = 1/2 * a * t^2
    | % % queda
    | % %    a = (v^2 - v0^2) / 2s
    | % %    t = ( v  -  v0 ) / a
    | % 
    | % % cmd.Fa = (vwp^2 - imu.ACvhor^2) / (2 * dis_hor);
    | % 
    | % 
    | % %calculo velocidad vertical
    | % if cmd.Fa == 0
    | %     % movimiento uniforme
    | %     t = dis_hor / imu.ACvhor;
    | % else
    | %     % movimiento uniformemente acelerado 
    | %     t = (vwp - imu.ACvhor) / cmd.Fa;
    | % end
    | % dist_vertical = cWP(3) - imu.ACz;
    | % cmd.Vs = dist_vertical / t;
    | % 
    | % 
    | % % if imu.ACy < 41000
    | % %     
    | % %     figure
    | % %     hold on
    | % %     grid on
    | % %     axis equal
    | % %     plot(cWP(1),cWP(2),'o')
    | % %     plot(imu.ACx,imu.ACy,'o')
    | % %     plot(cc(1),cc(2),'o')
    | % % end
    | 
    | 
    | 
    | end
    | 
    | 
    | 
    | 
    | 
    | 
    | function a = angulo(V1,V2)
    | % angulo para alcanzar desde V1 a V2
    | % sentido positivo contrario a las agujas del reloj
    | % angulo de salida (-180 +180]
    | 
    |     V1 = V1 / norm(V1);
    |     V2 = V2 / norm(V2);
    | 
    |     prod_esc = V1(1)*V2(1) + V1(2)*V2(2);
    |     if prod_esc > 1
    |         prod_esc = 1;
    |     end
    |     if prod_esc < -1
    |         prod_esc = -1;
    |     end
    |     a1 = acosd(prod_esc);
    | 
    |     prod_vec = V1(1)*V2(2) - V1(2)*V2(1);
    |     a2 = asind(prod_vec);
    |     
    |     a = a1*sign(a2);
    |     
    | end
  function sleep:
    | function sleep
    | 
    | % Desactivamos el avión y dejamos que pase un ciclo 
    | % ara que el RADAR lo elimine
    | ACenabled = 0;
    | 
    | ACoff.data = true;
    | send(ACoff);
  function ACmsgSend:
    | function ACmsgSend
    | 
    | ACmsg.data.ACid      = ACid;
    | ACmsg.data.ACenabled = ACenabled;
    | ACmsg.data.ACaborted = ACaborted;
    | 
    | ACmsg.data.ACx       = imu.ACx;
    | ACmsg.data.ACy       = imu.ACy;
    | ACmsg.data.ACz       = imu.ACz;
    | ACmsg.data.ACpsi     = imu.ACpsi;
    | ACmsg.data.ACvhor    = imu.ACvhor;
    | 
    | send(ACmsg)
  function abort = abortLanding:
    | function abort = abortLanding
    | % Decido si abortar el aterrizaje
    | % 
    | % persistent previously_aborted 
    | % if isempty(previously_aborted)
    | %     previously_aborted = false;
    | % end
    | 
    | abort = false;
    | 
    | if ACaborted
    |     return
    | end
    | 
    | if (ACid == 1) && (imu.ACz < 90) % DA/H: 295 ft (89.9 m)
    |     abort = true;
    |     ACaborted = 1;
    | end
  function updateRadar:
    | function updateRadar
    | 
    | radar.ACid      = ACid;
    | radar.ACenabled = ACenabled;
    | radar.ACdubins  = 1;
    | 
    | radar.ACx       = imu.ACx;
    | radar.ACy       = imu.ACy;
    | radar.ACz       = imu.ACz;
    | radar.ACpsi     = imu.ACpsi;
  function ATCmsgProcess:
    | function ATCmsgProcess
    | 
    | % extraigo informacion del mensaje
    | if ACenabled && ACid == ATCmsg.data.ACid
    |         cWP = [ATCmsg.data.WPx ATCmsg.data.WPy ATCmsg.data.WPz ATCmsg.data.WPspeed];
    | end
    | discard(ATCmsg)
    | 
    | %% Procesamiento del ATC

== stateflow chart AC/AC_Dubins_flyable/pilot ==
  state NAVIGATOR [parallel]
    settings: executionOrder=1
    state WAKEUP
      entry:
      wakeUp
      ACmsgSend
    state OFF
      entry:
      reset
    state SLEEP
      entry:
      sleep
      ACmsgSend
    state FLY
      entry, during:
      follow
      ACmsgSend
    (default) -> OFF
    OFF -> WAKEUP : [flightInfo.ACenabled]
    SLEEP -> OFF
    WAKEUP -> FLY
    FLY -> SLEEP : [landed]
  state COMUNICATIONS [parallel]
    updateRadar
    settings: executionOrder=2
  data: resp function_output; imuDubins input; cmdDubins input; imu input; cmd output Bus: bus_command; flightInfo input Bus: bus_ADSB; radar output Bus: bus_radar; ACid local double; cWP local; dist local; WP parameter; WPspeed parameter; ACenabled local; ACaborted local; ACmsg output Bus: bus_ACmsg
  function wakeUp:
    | function wakeUp
    | 
    | % inicializo navegación
    | ACid = flightInfo.ACid;
    | ACenabled = 1;
    | cWP = [WP(2,:) WPspeed(2)];
  function reset:
    | function reset
    | 
    | % reseteo estado de la aeronave
    | ACid = 0;
    | ACenabled = 0;
    | ACaborted = 0;
    | 
    | % reseteo movimiento
    | coder.extrinsic('convvel');
    | cmd.Fa = 123.4667; %convvel(cWP(4),'kts','m/s'); %123 m/s
    | cmd.Vs = 0;
    | cmd.Ys = 0;
  function resp = landed:
    | function resp = landed
    | % Concluye si el avion ha terminado de recorrer la pista
    | 
    | resp = false;
    | 
    | if imu.ACz < 50 % estamos a menos de 50 metros de altura
    |     %busco WP con velocidad 50 (solo el último la tiene)
    |     fWP = WP(find(WPspeed==50,1),:);
    |     %calculo segmento desde el AC a este WP
    |     s = fWP(1:2)-[imu.ACx imu.ACy];
    |     dist = norm(s);
    |     if dist < 50
    |         resp = true;
    |     end
    | end
  function sleep:
    | function sleep
    | 
    | % Desactivamos el avión y dejamos que pase un ciclo 
    | % ara que el RADAR lo elimine
    | ACenabled = 0;
  function follow:
    | function follow
    | 
    | p = [imuDubins.ACx-imu.ACx, imuDubins.ACy-imu.ACy];
    | 
    | alpha = imuDubins.ACpsi + cmdDubins.Ys;
    | F = [sin(alpha) cos(alpha)] * cmdDubins.Fa;
    | 
    | Fp = (F*60 + p) / 60;
    | cmd.Fa = norm(Fp);
    | alphap = atan2(Fp(1),Fp(2));
    |     
    | cmd.Ys = AngleBetweenOrientations(imu.ACpsi,alphap);
    | cmd.Ys = min(cmd.Ys,+0.05);
    | cmd.Ys = max(cmd.Ys,-0.05);
    | 
    | dz   = imuDubins.ACz - imu.ACz;    
    | kV  = 0.1;
    | varVs = kV * dz;
    | cmd.Vs = cmdDubins.Vs + varVs;
    | 
    | end
    | 
    | function a12 = AngleBetweenOrientations (or1,or2)
    | % ángulo mas corto desde la orientación or1 a la orientación or2
    | 
    |     or1 = rad2deg(or1);
    |     or1 = mod(or1,360);
    |  
    |     or2 = rad2deg(or2);
    |     or2 = mod(or2,360);
    | 
    |     a12 = or2-or1;
    | 
    |     if(a12 > 180)
    |         a12 = a12 - 360;
    |     end
    |     if(a12 < -180)
    |         a12 = a12 + 360;
    |     end
    | 
    |     a12 = deg2rad(a12);
    | end
  function ACmsgSend:
    | function ACmsgSend
    | 
    | ACmsg.data.ACid      = ACid;
    | ACmsg.data.ACenabled = 2; %ACenabled;
    | ACmsg.data.ACaborted = 0; %ACaborted;
    | 
    | ACmsg.data.ACx       = imu.ACx;
    | ACmsg.data.ACy       = imu.ACy;
    | ACmsg.data.ACz       = imu.ACz;
    | ACmsg.data.ACpsi     = imu.ACpsi;
    | ACmsg.data.ACvhor    = imu.ACvhor;
    | 
    | send(ACmsg)
  function updateRadar:
    | function updateRadar
    | 
    | radar.ACid      = ACid;
    | radar.ACenabled = ACenabled;
    | radar.ACdubins  = 0;
    | 
    | radar.ACx       = imu.ACx;
    | radar.ACy       = imu.ACy;
    | radar.ACz       = imu.ACz;
    | radar.ACpsi     = imu.ACpsi;
